simulink model "LAB07_1"  (R2022b)
settings: Solver=ode8  StartTime=0.0  StopTime=10000  FixedStep=0.05  RelTol=1e-3
values from neighbouring files (symbols this model uses):
  a = 6.843e6    (= 6843000)    [LAB_07_script.m]
  A0 = eye(3,3)    [LAB_07_script.m]
  e = 0.2    [LAB_07_script.m]
  epsilon = deg2rad(23.45)    [LAB_07_script.m]
  G = 6.6743e-11    [LAB_07_script.m]
  i = 0.1    [LAB_07_script.m]
  I = 10^-2*diag([100.9,25.1,91.6])    [LAB_07_script.m]
  Mt = 5.972e24    (= 5.972e+24)    [LAB_07_script.m]
  n = sqrt(G*Mt/R^3)    [LAB_07_script.m]
  n_sun = 2*pi/T_sun    (= 1.99238499086e-07)    [LAB_07_script.m]
  P = 1358/300000000    (= 4.52666666667e-06)    [LAB_07_script.m]
  position = 1e-2*[10,0,0;0,10,0;-10,0,0;0,-10,0;0,0,15;0,0,-15;0,45,0;0,45,0;0,-45,0;0,-45,0]    [LAB_07_script.m]
  R = 6.378e6    (= 6378000)    [LAB_07_script.m]
  r_sun = 149597870000    [LAB_07_script.m]
  rhoD_vector = ones(10,1)*0.1    [LAB_07_script.m]
  rhoS_vector = ones(10,1)*0.5    [LAB_07_script.m]
  rot_rate = 0.0012    [LAB_07_script.m]
  Surfaces_Matrix = [6e-2;6e-2;6e-2;6e-2;4e-2;4e-2;12e-2;12e-2;12e-2;12e-2]    [LAB_07_script.m]
  theta0 = 0    [LAB_07_script.m]
  Versor_Surfaces_Matrix = [  1   ,0  ,-1 ,0  ,0  ,0  ,1  ,-1 ,1  ,-1 ... (first row only)    [LAB_07_script.m]
  w0 = [0;0;n]    [LAB_07_script.m]
libraries: sharedutil x4, matrix_library x3
settings Model: Creator=ludov  LastModifiedBy=maria

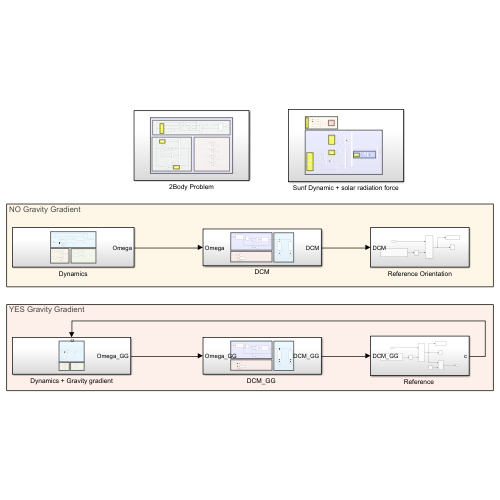
[thumbnail: Simulink's stored preview of the top-level diagram]
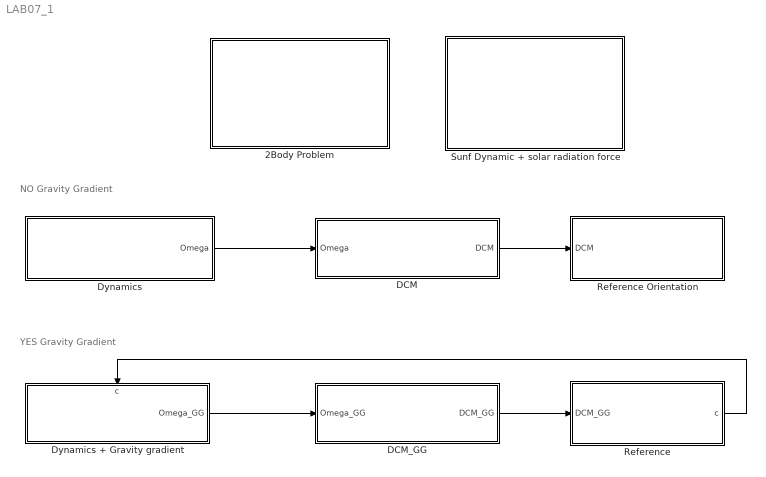
== system LAB07_1 ==
  note: NO Gravity Gradient
  note: YES Gravity Gradient
  2Body Problem : Subsystem
  DCM : Subsystem
  "DCM_GG " : Subsystem
  Dynamics : Subsystem
  Dynamics + Gravity gradient : Subsystem
      settings: PortSchema="{\"entries\":[{\"content\":{\"sides\":[{\"content\":{\"connectorIds\":[]},\"type\":\"ConnectorPlacement.EquallySpacedRectSide\",\"uuid\":\"36bea6c2-7c38-4cde-ba01-7aa966ff8266\"},{\"content\":{\"connectorIds\":[\"Out1\"],\"side\":\"RIGHT\"},\"type\":\"ConnectorPlacement.EquallySpacedRectSide\",\"uuid\":\"092edf66-02b8-469a-ae06-6e78e709ba5c\"},{\"content\":{\"connectorIds\":[\"In1\"],\"side\":\"TOP\"},\"type\":\"ConnectorPlacement.EquallySpacedRectSide\",\"uuid\":\"6c2573db-7f56-480a-a9c9-47590d2bcbd8\"},{\"content\":{\"connectorIds\":[],\"side\":\"BOTTOM\"},\"type\":\"ConnectorPlacement.EquallySpacedRectSide\",\"uuid\":\"1ca16e93-db1d-49db-8133-86d5d884b7d3\"}]},\"type\":\"ConnectorPlacement.EquallySpacedConnector\",\"uuid\":\"c0e06738-6361-48da-ae0d-4c1ab6a4c15e\"}],\"packageUris\":[\"http://schema.mathworks.com/mf0/Connector/R2020b\"],\"version\":\"1.0\"}"
  "Reference " : Subsystem
  Reference Orientation : Subsystem
  Sunf Dynamic + solar radiation force : Subsystem
  wires:
  DCM/1(DCM) -> Reference Orientation/1(DCM)
  Dynamics/1(Omega) -> DCM/1(Omega)
  "Reference "/1(c) -> Dynamics + Gravity gradient/1(c)
  "DCM_GG "/1(DCM_GG) -> "Reference "/1(DCM_GG)
  Dynamics + Gravity gradient/1(Omega_GG) -> "DCM_GG "/1(Omega_GG)

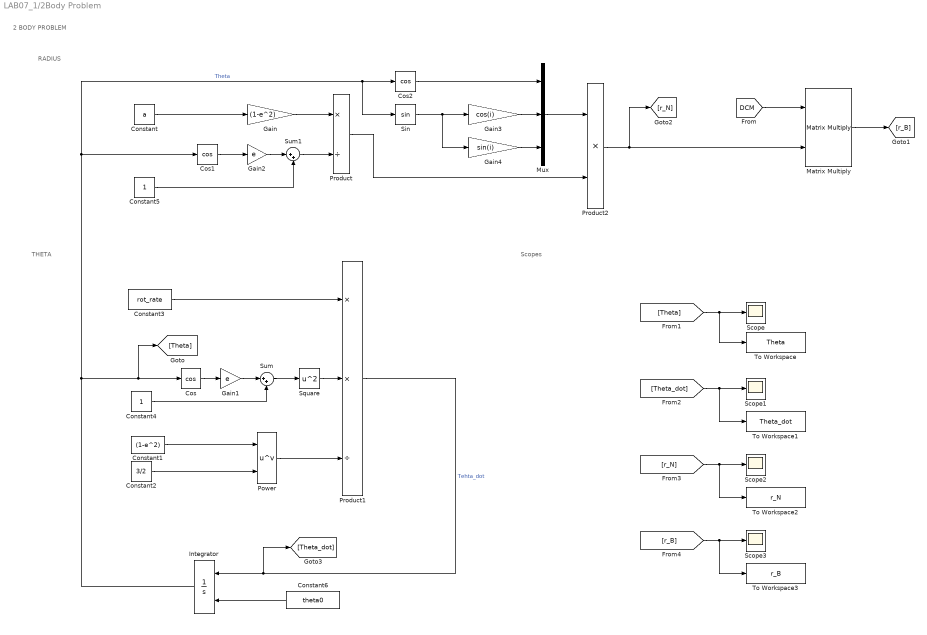
== system LAB07_1/2Body Problem ==
  note: RADIUS
  note: 2 BODY PROBLEM
  note: THETA
  note: Scopes
  Constant : Constant  Value=a
  Constant1 : Constant  Value=(1-e^2)
  Constant2 : Constant  Value=3/2
  Constant3 : Constant  Value=rot_rate
  Constant4 : Constant
  Constant5 : Constant
  Constant6 : Constant  Value=theta0
  Cos : Trigonometry  Operator=cos
  Cos1 : Trigonometry  Operator=cos
  Cos2 : Trigonometry  Operator=cos
  Gain : Gain  Gain=(1-e^2)
  Gain1 : Gain  Gain=e
  Gain2 : Gain  Gain=e
  Gain3 : Gain  Gain=cos(i)
  Gain4 : Gain  Gain=sin(i)
  Integrator : Integrator  InitialConditionSource=external  WrappedStateUpperValue=2*pi  WrappedStateLowerValue=0
  Matrix Multiply : Product  Multiplication=Matrix(*)
  Mux : Mux  Inputs=3
  Power : Math  Operator=pow
  Product : Product  Inputs=*/
  Product1 : Product  Inputs=**/
  Product2 : Product
  Scope{,1..3} (4 alike) : Scope
  Sin : Trigonometry
  Square : Math  Operator=square
  Sum : Sum  Inputs=|++
  Sum1 : Sum  Inputs=|++
  To Workspace : ToWorkspace  VariableName=Theta  SaveFormat=Timeseries  SampleTime=-1
  To Workspace1 : ToWorkspace  VariableName=Theta_dot  SaveFormat=Timeseries  SampleTime=-1
  To Workspace2 : ToWorkspace  VariableName=r_N  SaveFormat=Timeseries  SampleTime=-1
  To Workspace3 : ToWorkspace  VariableName=r_B  SaveFormat=Timeseries  SampleTime=-1
  wires:
  Constant/1 -> Gain/1
  Gain/1 -> Product/1
  Constant3/1 -> Product1/1
  Cos/1 -> Gain1/1
  Gain1/1 -> Sum/1
  Constant4/1 -> Sum/2
  Sum/1 -> Square/1
  Square/1 -> Product1/2
  Power/1 -> Product1/3
  Constant1/1 -> Power/1
  Constant2/1 -> Power/2
  Product1/1 -> [Theta_dot], Integrator/1  "Tehta_dot"
  Integrator/1 -> Cos2/1, Sin/1, Cos1/1, [Theta], Cos/1  "Theta"
  Cos1/1 -> Gain2/1
  Constant5/1 -> Sum1/2
  Gain2/1 -> Sum1/1
  Sum1/1 -> Product/2
  Constant6/1 -> Integrator/2
  Cos2/1 -> Mux/1
  Sin/1 -> Gain4/1, Gain3/1
  Gain3/1 -> Mux/2
  Gain4/1 -> Mux/3
  Mux/1 -> Product2/1
  Product/1 -> Product2/2
  Product2/1 -> [r_N], Matrix Multiply/2
  Matrix Multiply/1 -> [r_B]
  [DCM] -> Matrix Multiply/1
  [Theta_dot] -> To Workspace1/1, Scope1/1
  [Theta] -> To Workspace/1, Scope/1
  [r_N] -> To Workspace2/1, Scope2/1
  [r_B] -> To Workspace3/1, Scope3/1

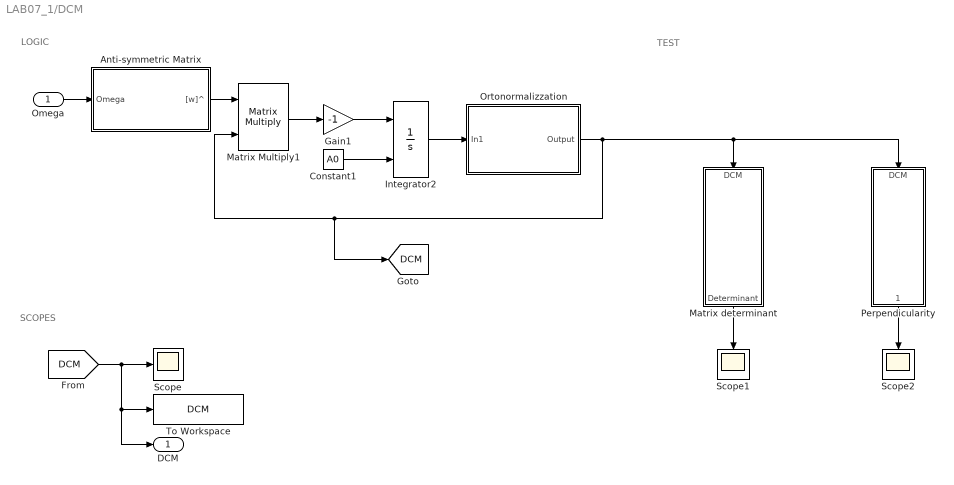
== system LAB07_1/DCM ==
  note: SCOPES
  note: LOGIC
  note: TEST
  Omega : Inport
  Anti-symmetric Matrix : Subsystem
  Constant1 : Constant  Value=A0
  Gain1 : Gain  Gain=-1
  Integrator2 : Integrator  InitialConditionSource=external
  Matrix Multiply1 : Product  Multiplication=Matrix(*)
  Matrix determinant : Subsystem
  Ortonormalizzation : Subsystem
  Perpendicularity : Subsystem
  Scope : Scope
  Scope1 : Scope
  Scope2 : Scope
  To Workspace : ToWorkspace  VariableName=DCM  SaveFormat=Timeseries  SampleTime=-1
  DCM : Outport
  tag scope: DCM=global
  wires:
  [DCM] -> DCM/1, To Workspace/1, Scope/1
  Anti-symmetric Matrix/1("[w]^") -> Matrix Multiply1/1
  Integrator2/1 -> Ortonormalizzation/1(In1)
  Matrix Multiply1/1 -> Gain1/1
  Ortonormalizzation/1(Output) -> Perpendicularity/1(DCM), Matrix determinant/1(DCM), Matrix Multiply1/2, [DCM]
  Omega/1 -> Anti-symmetric Matrix/1(Omega)
  Gain1/1 -> Integrator2/1
  Constant1/1 -> Integrator2/2
  Matrix determinant/1(Determinant) -> Scope1/1
  Perpendicularity/1(Perpendicularity flag) -> Scope2/1

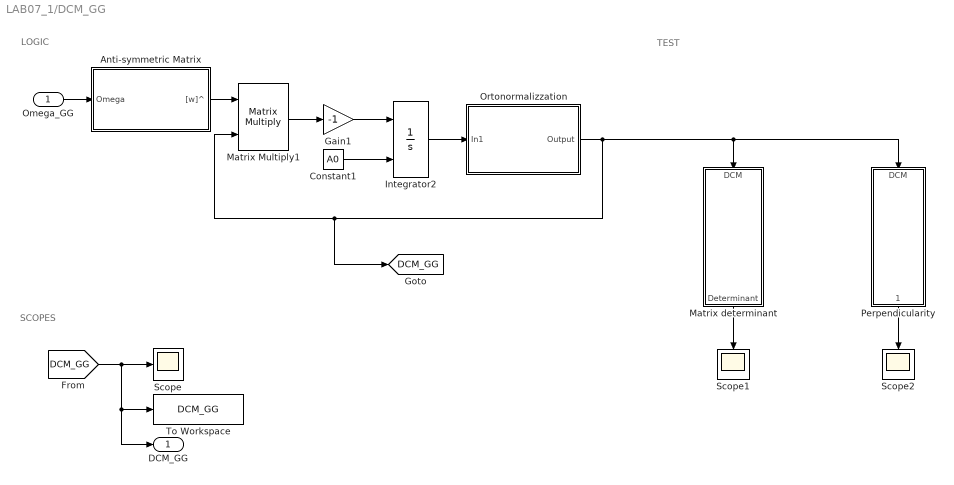
== system LAB07_1/DCM_GG  ==
  note: SCOPES
  note: LOGIC
  note: TEST
  Omega_GG : Inport
  Anti-symmetric Matrix : Subsystem
  Constant1 : Constant  Value=A0
  Gain1 : Gain  Gain=-1
  Integrator2 : Integrator  InitialConditionSource=external
  Matrix Multiply1 : Product  Multiplication=Matrix(*)
  Matrix determinant : Subsystem
  Ortonormalizzation : Subsystem
  Perpendicularity : Subsystem
  Scope : Scope
  Scope1 : Scope
  Scope2 : Scope
  To Workspace : ToWorkspace  VariableName=DCM_GG  SaveFormat=Timeseries  SampleTime=-1
  DCM_GG : Outport
  tag scope: DCM_GG=global
  wires:
  [DCM_GG] -> DCM_GG/1, To Workspace/1, Scope/1
  Anti-symmetric Matrix/1("[w]^") -> Matrix Multiply1/1
  Integrator2/1 -> Ortonormalizzation/1(In1)
  Matrix Multiply1/1 -> Gain1/1
  Ortonormalizzation/1(Output) -> Perpendicularity/1(DCM), Matrix determinant/1(DCM), Matrix Multiply1/2, [DCM_GG]
  Omega_GG/1 -> Anti-symmetric Matrix/1(Omega)
  Gain1/1 -> Integrator2/1
  Constant1/1 -> Integrator2/2
  Matrix determinant/1(Determinant) -> Scope1/1
  Perpendicularity/1(Perpendicularity flag) -> Scope2/1

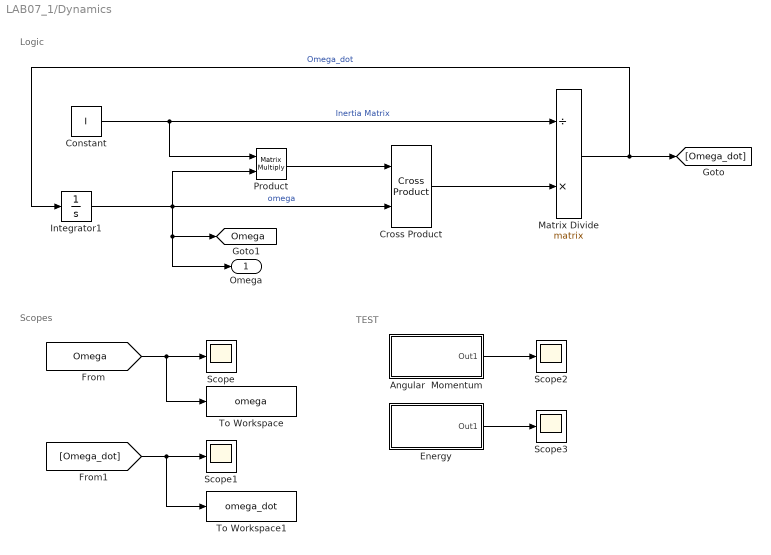
== system LAB07_1/Dynamics ==
  note: TEST
  note: Logic
  note: Scopes
  Angular  Momentum : Subsystem
  Constant : Constant  Value=I
  Cross Product : matrix_library/Cross Product
  Energy : Subsystem
  Integrator1 : Integrator  InitialCondition=w0
  Matrix Divide : Product  Inputs=/*  Multiplication=Matrix(*)
  Product : Product  Multiplication=Matrix(*)
  Scope{,1..3} (4 alike) : Scope
  To Workspace : ToWorkspace  VariableName=omega  SaveFormat=Timeseries  SampleTime=-1
  To Workspace1 : ToWorkspace  VariableName=omega_dot  SaveFormat=Timeseries  SampleTime=-1
  Omega : Outport
  tag scope: Omega=global
  wires:
  Product/1 -> Cross Product/1
  Integrator1/1 -> Cross Product/2, Product/2, Omega/1, [Omega]  "omega"
  Matrix Divide/1 -> [Omega_dot], Integrator1/1  "Omega_dot"
  Constant/1 -> Product/1, Matrix Divide/1  "Inertia Matrix"
  Cross Product/1 -> Matrix Divide/2
  [Omega] -> To Workspace/1, Scope/1
  [Omega_dot] -> To Workspace1/1, Scope1/1
  Angular  Momentum/1(Out1) -> Scope2/1
  Energy/1(Out1) -> Scope3/1

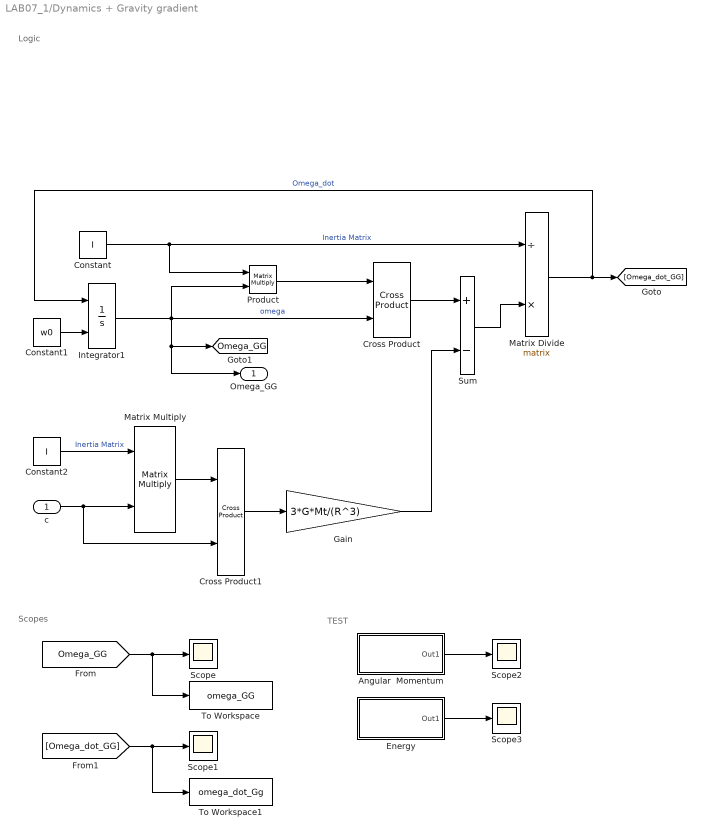
== system LAB07_1/Dynamics + Gravity gradient ==
  note: TEST
  note: Scopes
  note: Logic
  c : Inport
  Angular  Momentum : Subsystem
  Constant : Constant  Value=I
  Constant1 : Constant  Value=w0
  Constant2 : Constant  Value=I
  Cross Product : matrix_library/Cross Product
  Cross Product1 : matrix_library/Cross Product
  Energy : Subsystem
  Gain : Gain  Gain=3*G*Mt/(R^3)
  Integrator1 : Integrator  InitialConditionSource=external  InitialCondition=w0
  Matrix Divide : Product  Inputs=/*  Multiplication=Matrix(*)
  Matrix Multiply : Product  Multiplication=Matrix(*)
  Product : Product  Multiplication=Matrix(*)
  Scope{,1..3} (4 alike) : Scope
  Sum : Sum  Inputs=+-
  To Workspace : ToWorkspace  VariableName=omega_GG  SaveFormat=Timeseries  SampleTime=-1
  To Workspace1 : ToWorkspace  VariableName=omega_dot_Gg  SaveFormat=Timeseries  SampleTime=-1
  Omega_GG : Outport
  tag scope: Omega_GG=global
  wires:
  [Omega_dot_GG] -> To Workspace1/1, Scope1/1
  [Omega_GG] -> To Workspace/1, Scope/1
  Integrator1/1 -> Omega_GG/1, [Omega_GG], Cross Product/2, Product/2  "omega"
  Matrix Divide/1 -> Integrator1/1, [Omega_dot_GG]  "Omega_dot"
  Constant/1 -> Product/1, Matrix Divide/1  "Inertia Matrix"
  Energy/1(Out1) -> Scope3/1
  Angular  Momentum/1(Out1) -> Scope2/1
  Product/1 -> Cross Product/1
  Cross Product/1 -> Sum/1
  Sum/1 -> Matrix Divide/2
  Constant1/1 -> Integrator1/2
  c/1 -> Matrix Multiply/2, Cross Product1/2
  Constant2/1 -> Matrix Multiply/1  "Inertia Matrix"
  Matrix Multiply/1 -> Cross Product1/1
  Cross Product1/1 -> Gain/1
  Gain/1 -> Sum/2

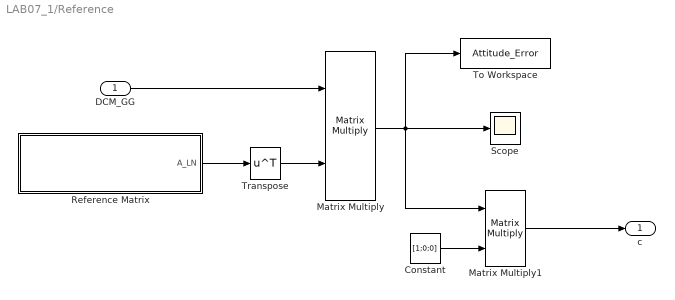
== system LAB07_1/Reference  ==
  DCM_GG : Inport
  Constant : Constant  Value=[1;0;0]
  Matrix Multiply : Product  Multiplication=Matrix(*)
  Matrix Multiply1 : Product  Multiplication=Matrix(*)
  Reference Matrix : Subsystem
  Scope : Scope
  To Workspace : ToWorkspace  VariableName=Attitude_Error  SampleTime=-1
  Transpose : Math  Operator=transpose
  c : Outport
  wires:
  Transpose/1 -> Matrix Multiply/2
  Reference Matrix/1(A_LN) -> Transpose/1
  Matrix Multiply/1 -> Matrix Multiply1/1, Scope/1, To Workspace/1
  DCM_GG/1 -> Matrix Multiply/1
  Constant/1 -> Matrix Multiply1/2
  Matrix Multiply1/1 -> c/1

== system LAB07_1/Reference Orientation ==
  DCM : Inport
  Matrix Multiply : Product  Multiplication=Matrix(*)
  Reference Matrix : Subsystem
  Scope : Scope
  To Workspace : ToWorkspace  VariableName=err  SampleTime=-1
  Transpose : Math  Operator=transpose
  wires:
  Transpose/1 -> Matrix Multiply/2
  Reference Matrix/1(A_LN) -> Transpose/1
  Matrix Multiply/1 -> To Workspace/1, Scope/1
  DCM/1 -> Matrix Multiply/1

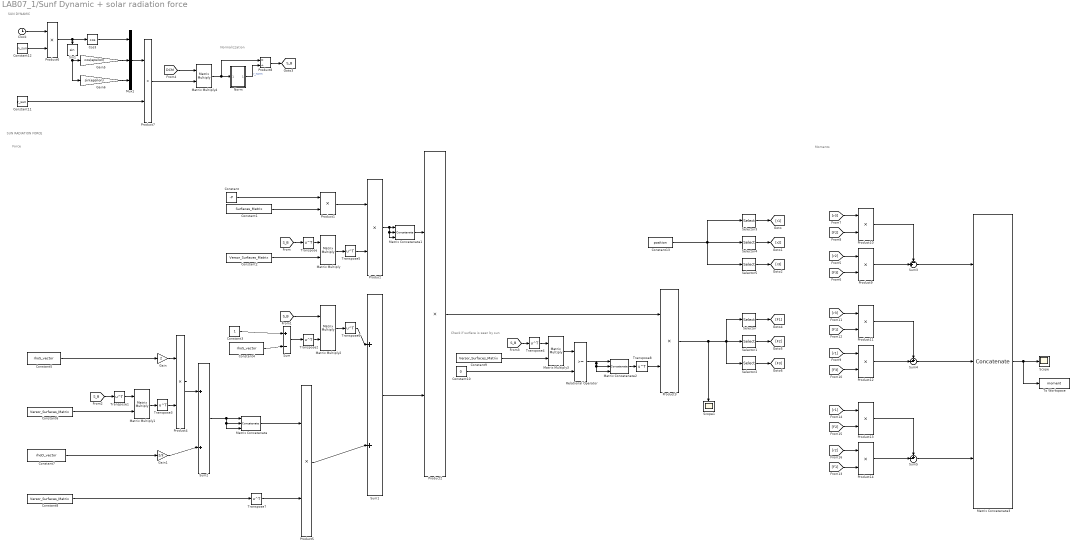
== system LAB07_1/Sunf Dynamic + solar radiation force ==
  note: Moments
  note: Force
  note: Check if surface is seen by sun
  note: SUN RADIATION FORCE
  note: Normalizzation
  note: SUN DYNAMIC
  Clock : Clock
  Constant : Constant  Value=-P
  Constant1 : Constant  Value=Surfaces_Matrix
  Constant10 : Constant  Value=0
  Constant11 : Constant  Value=r_sun
  Constant12 : Constant  Value=n_sun
  Constant13 : Constant  Value=position
  Constant{2,6,8..9} (4 alike) : Constant  Value=Versor_Surfaces_Matrix
  Constant3 : Constant
  Constant4 : Constant  Value=rhoS_vector
  Constant5 : Constant  Value=rhoS_vector
  Constant7 : Constant  Value=rhoD_vector
  Cos3 : Trigonometry  Operator=cos
  Gain : Gain  Gain=2
  Gain1 : Gain  Gain=2/3
  Gain5 : Gain  Gain=cos(epsilon)
  Gain6 : Gain  Gain=sin(epsilon)
  Matrix Concatenate : Concatenate  NumInputs=3  Mode=Multidimensional array  ConcatenateDimension=2
  Matrix Concatenate1 : Concatenate  NumInputs=3  Mode=Multidimensional array  ConcatenateDimension=2
  Matrix Concatenate2 : Concatenate  NumInputs=3  Mode=Multidimensional array
  Matrix Concatenate3 : Concatenate  NumInputs=3  Mode=Multidimensional array  ConcatenateDimension=2
  Matrix Multiply{,1..4} (5 alike) : Product  Multiplication=Matrix(*)
  Mux1 : Mux  Inputs=3
  Norm : Subsystem
  Product{,1..7,9..14} (14 alike) : Product
  Product8 : Product  Inputs=*/
  Relational Operator : RelationalOperator  OutDataTypeStr=boolean  RndMeth=Simplest  InputSameDT=off
  Scope : Scope
  Scope1 : Scope
  Selector : Selector  NumberOfDimensions=2  InputPortWidth=3  IndexOptions=Select all,Index vector (dialog)  Indices=1,1  OutputSizes=1,1
  Selector1 : Selector  NumberOfDimensions=2  InputPortWidth=3  IndexOptions=Select all,Index vector (dialog)  Indices=1,2  OutputSizes=1,1
  Selector2 : Selector  NumberOfDimensions=2  InputPortWidth=3  IndexOptions=Select all,Index vector (dialog)  Indices=1,3  OutputSizes=1,1
  Selector3 : Selector  NumberOfDimensions=2  InputPortWidth=3  IndexOptions=Select all,Index vector (dialog)  Indices=1,1  OutputSizes=1,1
  Selector4 : Selector  NumberOfDimensions=2  InputPortWidth=3  IndexOptions=Select all,Index vector (dialog)  Indices=1,2  OutputSizes=1,1
  Selector5 : Selector  NumberOfDimensions=2  InputPortWidth=3  IndexOptions=Select all,Index vector (dialog)  Indices=1,3  OutputSizes=1,1
  Sin1 : Trigonometry
  Sum : Sum  Inputs=+|-
  Sum1 : Sum  Inputs=+|+
  Sum2 : Sum  Inputs=+|+
  Sum3 : Sum  Inputs=-+|
  Sum4 : Sum  Inputs=+-|
  Sum5 : Sum  Inputs=+-|
  To Workspace : ToWorkspace  VariableName=moment  SampleTime=-1
  Transpose{,1..8} (9 alike) : Math  Operator=transpose
  tag scope: S_B=global
  wires:
  Constant/1 -> Product1/1
  Product1/1 -> Product/1
  Constant1/1 -> Product1/2
  Matrix Multiply/1 -> Transpose5/1
  [S_B] -> Transpose/1
  Constant2/1 -> Matrix Multiply/2
  [S_B] -> Matrix Multiply2/1
  Constant3/1 -> Sum/1
  Constant4/1 -> Sum/2
  Transpose/1 -> Matrix Multiply/1
  Constant5/1 -> Gain/1
  [S_B] -> Transpose1/1
  Constant6/1 -> Matrix Multiply1/2
  Matrix Multiply1/1 -> Transpose3/1
  Gain/1 -> Product4/1
  Constant7/1 -> Gain1/1
  Matrix Multiply2/1 -> Transpose6/1
  Sum/1 -> Transpose2/1
  Transpose2/1 -> Matrix Multiply2/2
  Gain1/1 -> Sum2/2
  Transpose5/1 -> Product/2
  Product4/1 -> Sum2/1
  Transpose1/1 -> Matrix Multiply1/1
  Transpose3/1 -> Product4/2
  Product5/1 -> Sum1/2
  Transpose6/1 -> Sum1/1
  Constant8/1 -> Transpose7/1
  Transpose7/1 -> Product5/2
  Sum2/1 -> Matrix Concatenate/3, Matrix Concatenate/2, Matrix Concatenate/1
  Matrix Concatenate/1 -> Product5/1
  Product/1 -> Matrix Concatenate1/3, Matrix Concatenate1/2, Matrix Concatenate1/1
  Matrix Concatenate1/1 -> Product2/1
  Constant10/1 -> Relational Operator/2
  Sum1/1 -> Product2/2
  [S_B] -> Transpose4/1
  Matrix Multiply3/1 -> Relational Operator/1
  Transpose4/1 -> Matrix Multiply3/1
  Constant9/1 -> Matrix Multiply3/2
  Relational Operator/1 -> Matrix Concatenate2/3, Matrix Concatenate2/2, Matrix Concatenate2/1
  Matrix Concatenate2/1 -> Transpose8/1
  Product2/1 -> Product3/1
  Transpose8/1 -> Product3/2
  Product3/1 -> Selector/1, Selector2/1, Selector1/1, Scope1/1
  Sin1/1 -> Gain6/1, Gain5/1
  Gain6/1 -> Mux1/3
  Norm/1(Out1) -> Product8/2  "r_norm"
  Product8/1 -> [S_B]
  Cos3/1 -> Mux1/1
  Constant11/1 -> Product7/2
  Constant12/1 -> Product6/2
  Matrix Multiply4/1 -> Product8/1, Norm/1(In1)
  Product6/1 -> Sin1/1, Cos3/1
  Mux1/1 -> Product7/1
  [DCM] -> Matrix Multiply4/1
  Clock/1 -> Product6/1
  Gain5/1 -> Mux1/2
  Product7/1 -> Matrix Multiply4/2
  Constant13/1 -> Selector5/1, Selector4/1, Selector3/1
  Selector3/1 -> [r1]
  Selector4/1 -> [r2]
  Selector5/1 -> [r3]
  Selector/1 -> [F1]
  Selector1/1 -> [F2]
  Selector2/1 -> [F3]
  [r2] -> Product9/1
  [F3] -> Product9/2
  Product9/1 -> Sum3/2
  [F2] -> Product10/2
  [r3] -> Product10/1
  Product10/1 -> Sum3/1
  Product12/1 -> Sum4/2
  [F3] -> Product12/2
  [r1] -> Product12/1
  [r3] -> Product11/1
  [F1] -> Product11/2
  Product11/1 -> Sum4/1
  Product14/1 -> Sum5/2
  [F1] -> Product14/2
  Product13/1 -> Sum5/1
  [r2] -> Product14/1
  [F2] -> Product13/2
  [r1] -> Product13/1
  Sum5/1 -> Matrix Concatenate3/3
  Sum4/1 -> Matrix Concatenate3/2
  Sum3/1 -> Matrix Concatenate3/1
  Matrix Concatenate3/1 -> Scope/1, To Workspace/1

== system LAB07_1/DCM/Anti-symmetric Matrix ==
  Omega : Inport
  Demux : Demux  Outputs=3
  Gain : Gain  Gain=[0,0,0;0,0,-1;0,1,0]
  Gain1 : Gain  Gain=[0,0,1;0,0,0;-1,0,0]
  Gain2 : Gain  Gain=[0,-1,0;1,0,0;0,0,0]
  Sum : Sum  Inputs=+++
  "[w]^" : Outport
  wires:
  Sum/1 -> "[w]^"/1
  Demux/1 -> Gain/1
  Gain/1 -> Sum/1
  Demux/3 -> Gain2/1
  Gain2/1 -> Sum/3
  Demux/2 -> Gain1/1
  Gain1/1 -> Sum/2
  Omega/1 -> Demux/1

== system LAB07_1/DCM/Matrix determinant ==
  DCM : Inport
  Determinant of 3x3 Matrix : sharedutil/Determinant of 3x3 Matrix  aMode=aMode
      settings: LibrarySourceBlock=|
      | aerolibutil/Determinant of
      | 3x3 Matrix
  Determinant : Outport
  wires:
  Determinant of 3x3 Matrix/1 -> Determinant/1
  DCM/1 -> Determinant of 3x3 Matrix/1

== system LAB07_1/DCM/Ortonormalizzation ==
  In1 : Inport
  Gain : Gain  Gain=1.5
  Gain1 : Gain  Gain=0.5
  Matrix Multiply : Product  Inputs=3  Multiplication=Matrix(*)
  Sum : Sum  Inputs=|+-
  Transpose : Math  Operator=transpose
  Output : Outport
  wires:
  Matrix Multiply/1 -> Gain1/1
  Gain/1 -> Sum/1
  In1/1 -> Matrix Multiply/3, Gain/1, Transpose/1, Matrix Multiply/1
  Gain1/1 -> Sum/2
  Transpose/1 -> Matrix Multiply/2
  Sum/1 -> Output/1

== system LAB07_1/DCM/Perpendicularity ==
  DCM : Inport
  MATLAB Function2 : MATLAB Function  TreatAsAtomicUnit=on
  Perpendicularity flag : Outport
  wires:
  MATLAB Function2/1(perpendicularity_flag) -> Perpendicularity flag/1
  DCM/1 -> MATLAB Function2/1(DCM)

== system LAB07_1/DCM_GG /Anti-symmetric Matrix ==
  Omega : Inport
  Demux : Demux  Outputs=3
  Gain : Gain  Gain=[0,0,0;0,0,-1;0,1,0]
  Gain1 : Gain  Gain=[0,0,1;0,0,0;-1,0,0]
  Gain2 : Gain  Gain=[0,-1,0;1,0,0;0,0,0]
  Sum : Sum  Inputs=+++
  "[w]^" : Outport
  wires:
  Sum/1 -> "[w]^"/1
  Demux/1 -> Gain/1
  Gain/1 -> Sum/1
  Demux/3 -> Gain2/1
  Gain2/1 -> Sum/3
  Demux/2 -> Gain1/1
  Gain1/1 -> Sum/2
  Omega/1 -> Demux/1

== system LAB07_1/DCM_GG /Matrix determinant ==
  DCM : Inport
  Determinant of 3x3 Matrix : sharedutil/Determinant of 3x3 Matrix  aMode=aMode
      settings: LibrarySourceBlock=|
      | aerolibutil/Determinant of
      | 3x3 Matrix
  Determinant : Outport
  wires:
  Determinant of 3x3 Matrix/1 -> Determinant/1
  DCM/1 -> Determinant of 3x3 Matrix/1

== system LAB07_1/DCM_GG /Ortonormalizzation ==
  In1 : Inport
  Gain : Gain  Gain=1.5
  Gain1 : Gain  Gain=0.5
  Matrix Multiply : Product  Inputs=3  Multiplication=Matrix(*)
  Sum : Sum  Inputs=|+-
  Transpose : Math  Operator=transpose
  Output : Outport
  wires:
  Matrix Multiply/1 -> Gain1/1
  Gain/1 -> Sum/1
  In1/1 -> Matrix Multiply/3, Gain/1, Transpose/1, Matrix Multiply/1
  Gain1/1 -> Sum/2
  Transpose/1 -> Matrix Multiply/2
  Sum/1 -> Output/1

== system LAB07_1/DCM_GG /Perpendicularity ==
  DCM : Inport
  MATLAB Function2 : MATLAB Function  TreatAsAtomicUnit=on
  Perpendicularity flag : Outport
  wires:
  MATLAB Function2/1(perpendicularity_flag) -> Perpendicularity flag/1
  DCM/1 -> MATLAB Function2/1(DCM)

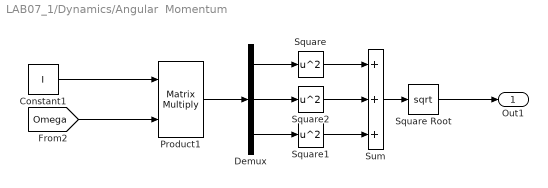
== system LAB07_1/Dynamics/Angular  Momentum ==
  Constant1 : Constant  Value=I
  Demux : Demux  Outputs=3
  Product1 : Product  Multiplication=Matrix(*)
  Square : Math  Operator=square
  Square Root : Sqrt
  Square1 : Math  Operator=square
  Square2 : Math  Operator=square
  Sum : Sum  Inputs=+++
  Out1 : Outport
  wires:
  [Omega] -> Product1/2
  Constant1/1 -> Product1/1
  Product1/1 -> Demux/1
  Square Root/1 -> Out1/1
  Demux/1 -> Square/1
  Demux/2 -> Square2/1
  Demux/3 -> Square1/1
  Square/1 -> Sum/1
  Square2/1 -> Sum/2
  Square1/1 -> Sum/3
  Sum/1 -> Square Root/1

== system LAB07_1/Dynamics/Energy ==
  Constant1 : Constant  Value=I
  Gain : Gain  Gain=0.5
  Matrix Multiply : Product  Multiplication=Matrix(*)
  Matrix Multiply1 : Product  Multiplication=Matrix(*)
  Transpose : Math  Operator=transpose
  Out1 : Outport
  wires:
  Matrix Multiply1/1 -> Gain/1
  Matrix Multiply/1 -> Matrix Multiply1/1
  [Omega] -> Matrix Multiply1/2, Transpose/1
  Transpose/1 -> Matrix Multiply/1
  Gain/1 -> Out1/1
  Constant1/1 -> Matrix Multiply/2

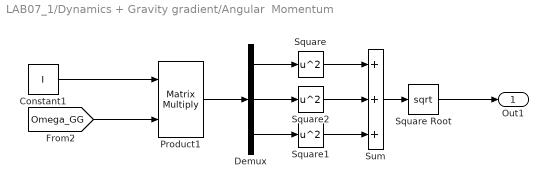
== system LAB07_1/Dynamics + Gravity gradient/Angular  Momentum ==
  Constant1 : Constant  Value=I
  Demux : Demux  Outputs=3
  Product1 : Product  Multiplication=Matrix(*)
  Square : Math  Operator=square
  Square Root : Sqrt
  Square1 : Math  Operator=square
  Square2 : Math  Operator=square
  Sum : Sum  Inputs=+++
  Out1 : Outport
  wires:
  [Omega_GG] -> Product1/2
  Constant1/1 -> Product1/1
  Product1/1 -> Demux/1
  Square Root/1 -> Out1/1
  Demux/1 -> Square/1
  Demux/2 -> Square2/1
  Demux/3 -> Square1/1
  Square/1 -> Sum/1
  Square2/1 -> Sum/2
  Square1/1 -> Sum/3
  Sum/1 -> Square Root/1

== system LAB07_1/Dynamics + Gravity gradient/Energy ==
  Constant1 : Constant  Value=I
  Gain : Gain  Gain=0.5
  Matrix Multiply : Product  Multiplication=Matrix(*)
  Matrix Multiply1 : Product  Multiplication=Matrix(*)
  Transpose : Math  Operator=transpose
  Out1 : Outport
  wires:
  Matrix Multiply1/1 -> Gain/1
  Matrix Multiply/1 -> Matrix Multiply1/1
  [Omega_GG] -> Matrix Multiply1/2, Transpose/1
  Transpose/1 -> Matrix Multiply/1
  Gain/1 -> Out1/1
  Constant1/1 -> Matrix Multiply/2

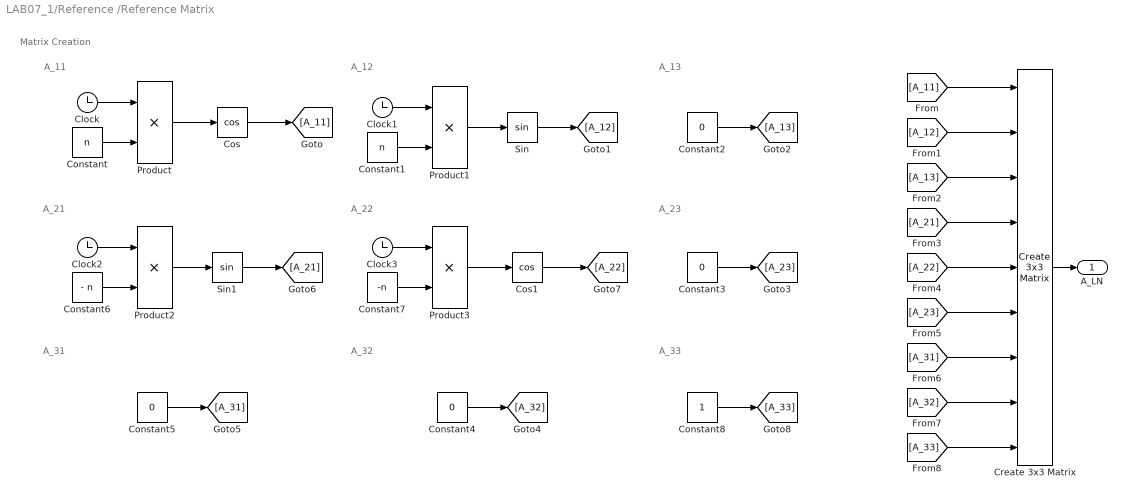
== system LAB07_1/Reference /Reference Matrix ==
  note: Matrix Creation
  note: A_11
  note: A_12
  note: A_13
  note: A_23
  note: A_33
  note: A_22
  note: A_21
  note: A_31
  note: A_32
  Clock{,1..3} (4 alike) : Clock
  Constant : Constant  Value=n
  Constant1 : Constant  Value=n
  Constant{2..5} (4 alike) : Constant  Value=0
  Constant6 : Constant  Value=- n  VectorParams1D=off
  Constant7 : Constant  Value=-n
  Constant8 : Constant
  Cos : Trigonometry  Operator=cos
  Cos1 : Trigonometry  Operator=cos
  Create 3x3 Matrix : sharedutil/Create 3x3 Matrix  aMode=aMode
      settings: LibrarySourceBlock=aerolibutil/Create 3x3 Matrix
  Product{,1..3} (4 alike) : Product
  Sin : Trigonometry
  Sin1 : Trigonometry
  A_LN : Outport
  wires:
  Clock/1 -> Product/1
  Constant/1 -> Product/2
  Product/1 -> Cos/1
  Cos/1 -> [A_11]
  Product1/1 -> Sin/1
  Constant1/1 -> Product1/2
  Clock1/1 -> Product1/1
  Sin/1 -> [A_12]
  Constant2/1 -> [A_13]
  Constant3/1 -> [A_23]
  Constant4/1 -> [A_32]
  Constant5/1 -> [A_31]
  Sin1/1 -> [A_21]
  Product2/1 -> Sin1/1
  Constant6/1 -> Product2/2
  Clock2/1 -> Product2/1
  Product3/1 -> Cos1/1
  Constant7/1 -> Product3/2
  Cos1/1 -> [A_22]
  Clock3/1 -> Product3/1
  Constant8/1 -> [A_33]
  [A_11] -> Create 3x3 Matrix/1
  [A_12] -> Create 3x3 Matrix/2
  [A_13] -> Create 3x3 Matrix/3
  [A_21] -> Create 3x3 Matrix/4
  [A_22] -> Create 3x3 Matrix/5
  [A_23] -> Create 3x3 Matrix/6
  [A_31] -> Create 3x3 Matrix/7
  [A_32] -> Create 3x3 Matrix/8
  [A_33] -> Create 3x3 Matrix/9
  Create 3x3 Matrix/1 -> A_LN/1

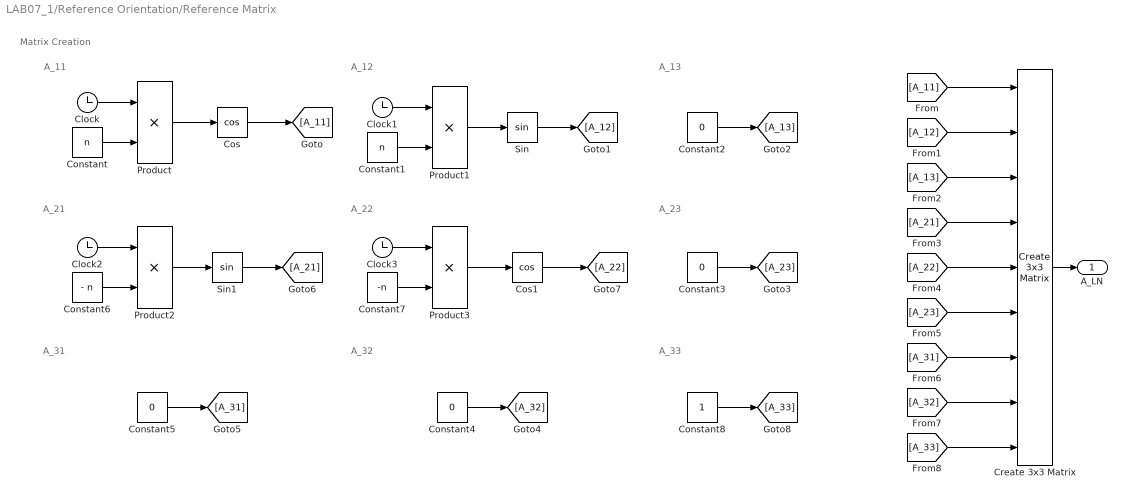
== system LAB07_1/Reference Orientation/Reference Matrix ==
  note: Matrix Creation
  note: A_11
  note: A_12
  note: A_13
  note: A_23
  note: A_33
  note: A_22
  note: A_21
  note: A_31
  note: A_32
  Clock{,1..3} (4 alike) : Clock
  Constant : Constant  Value=n
  Constant1 : Constant  Value=n
  Constant{2..5} (4 alike) : Constant  Value=0
  Constant6 : Constant  Value=- n  VectorParams1D=off
  Constant7 : Constant  Value=-n
  Constant8 : Constant
  Cos : Trigonometry  Operator=cos
  Cos1 : Trigonometry  Operator=cos
  Create 3x3 Matrix : sharedutil/Create 3x3 Matrix  aMode=aMode
      settings: LibrarySourceBlock=aerolibutil/Create 3x3 Matrix
  Product{,1..3} (4 alike) : Product
  Sin : Trigonometry
  Sin1 : Trigonometry
  A_LN : Outport
  wires:
  Clock/1 -> Product/1
  Constant/1 -> Product/2
  Product/1 -> Cos/1
  Cos/1 -> [A_11]
  Product1/1 -> Sin/1
  Constant1/1 -> Product1/2
  Clock1/1 -> Product1/1
  Sin/1 -> [A_12]
  Constant2/1 -> [A_13]
  Constant3/1 -> [A_23]
  Constant4/1 -> [A_32]
  Constant5/1 -> [A_31]
  Sin1/1 -> [A_21]
  Product2/1 -> Sin1/1
  Constant6/1 -> Product2/2
  Clock2/1 -> Product2/1
  Product3/1 -> Cos1/1
  Constant7/1 -> Product3/2
  Cos1/1 -> [A_22]
  Clock3/1 -> Product3/1
  Constant8/1 -> [A_33]
  [A_11] -> Create 3x3 Matrix/1
  [A_12] -> Create 3x3 Matrix/2
  [A_13] -> Create 3x3 Matrix/3
  [A_21] -> Create 3x3 Matrix/4
  [A_22] -> Create 3x3 Matrix/5
  [A_23] -> Create 3x3 Matrix/6
  [A_31] -> Create 3x3 Matrix/7
  [A_32] -> Create 3x3 Matrix/8
  [A_33] -> Create 3x3 Matrix/9
  Create 3x3 Matrix/1 -> A_LN/1

== system LAB07_1/Sunf Dynamic + solar radiation force/Norm ==
  In1 : Inport
  Demux : Demux  Outputs=3
  Square : Math  Operator=square
  Square Root : Sqrt
  Square1 : Math  Operator=square
  Square2 : Math  Operator=square
  Sum : Sum  Inputs=+++
  Out1 : Outport
  wires:
  Demux/3 -> Square2/1
  Sum/1 -> Square Root/1
  Demux/1 -> Square/1
  Square1/1 -> Sum/2
  Demux/2 -> Square1/1
  In1/1 -> Demux/1
  Square2/1 -> Sum/3
  Square/1 -> Sum/1
  Square Root/1 -> Out1/1

== matlab function LAB07_1/DCM/Perpendicularity/MATLAB Function2 ==
  data: DCM input; perpendicularity_flag output
function perpendicularity_flag = fcn(DCM)
    

perpendicularity_flag =zeros(3,1);

    x   = DCM(1,:);
    y   = DCM(2,:);
    z   = DCM(3,:);

    perpendicularity_flag(1)=dot(x,y);
    perpendicularity_flag(2)=dot(x,z);
    perpendicularity_flag(3)=dot(z,y);

end

== matlab function LAB07_1/DCM_GG /Perpendicularity/MATLAB Function2 ==
  data: DCM input; perpendicularity_flag output
function perpendicularity_flag = fcn(DCM)
    

perpendicularity_flag =zeros(3,1);

    x   = DCM(1,:);
    y   = DCM(2,:);
    z   = DCM(3,:);

    perpendicularity_flag(1)=dot(x,y);
    perpendicularity_flag(2)=dot(x,z);
    perpendicularity_flag(3)=dot(z,y);

end
